simulink model "sim_main_esb_14"  (R2019b)
settings: Solver=VariableStepAuto  StartTime=0.0  StopTime=1  RelTol=1e-3
values from neighbouring files (symbols this model uses):
  C = 0.344    [KALMAN.m]    (also in main_sys.m = double( subs( C) ); main_sys_klm.m = double( subs( C) ); main_tf_0.m = [ 0 , 0  , Ks , ds , -Ks , -ds, 0 ]; main_tf_1.m = C_mes)
  Ct = double( subs( Ct) )    [main_sys.m]    (also in main_sys_klm.m; main_tf_10.m; main_tf_11.m; main_tf_12.m)
  sys_sys = ss(A,B,C,D)    [main_sys.m]    (also in main_sys_klm.m; main_tf_10.m; main_tf_11.m; main_tf_12.m = ss(A_sys,B_sys,C_sys_mod,D_sys_mod))
  Trq_mot_nom = .56    (= 0.56)    [main_cntl.m]    (also in main_sys.m; main_sys_klm.m; main_tf_10.m; main_tf_11.m)
  Tsk = .001    (= 0.001)    [main_tf_11.m]    (also in main_tf_12.m; main_tf_13.m)
  v_trq = 35e-3    (= 0.035)    [main_tf_11.m]    (also in main_tf_12.m; main_tf_13.m)
  v_vel = .1e-6    (= 1e-07)    [main_tf_11.m]    (also in main_tf_12.m; main_tf_13.m)
  w_trq = .1e-3    (= 0.0001)    [main_tf_11.m]    (also in main_tf_12.m; main_tf_13.m)
  w_vel = .15e-3    (= 0.00015)    [main_tf_11.m]    (also in main_tf_12.m; main_tf_13.m)
undefined symbols (not defined in the file or in its folder): Discrete, K_lq3, Time
libraries: ctrlSharedLib x1
settings Model: Creator=eshojaei  LastModifiedBy=eshojaei
settings DataIOCC: ReturnWorkspaceOutputs=off
settings DebuggingCC: ArithmeticOperatorsInVariantConditions=warning
settings SFSimCC: CustomCodeUndefinedFunction=UseInterfaceOnly
settings CodeAppCC: StateflowObjectComments=on

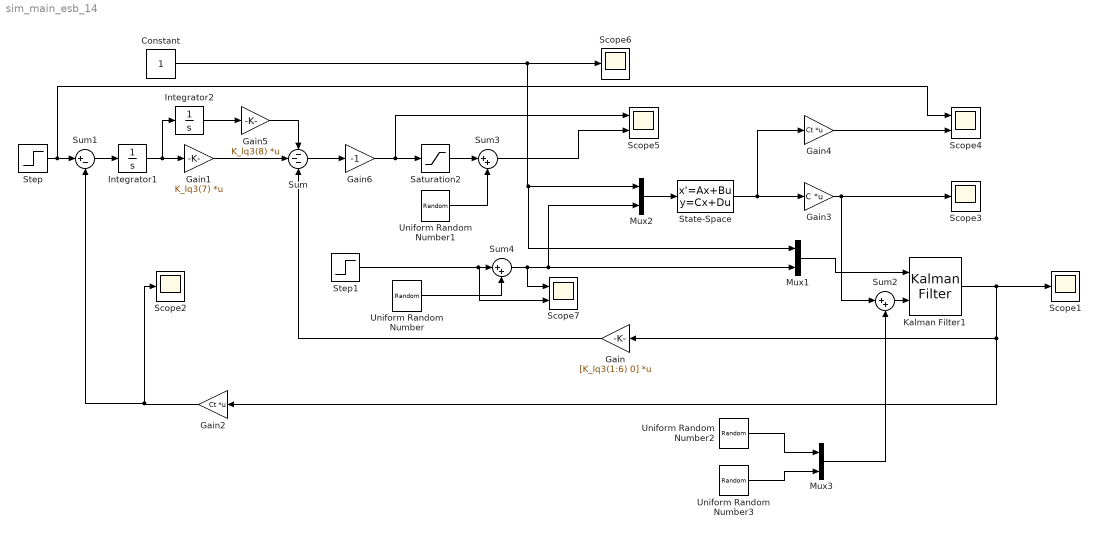
== system sim_main_esb_14 ==
  Constant : Constant
  Gain : Gain  Gain=[K_lq3(1:6) 0]  Multiplication=Matrix(K*u)
  Gain1 : Gain  Gain=K_lq3(7)  Multiplication=Matrix(K*u)
  Gain2 : Gain  Gain=Ct  Multiplication=Matrix(K*u)
  Gain3 : Gain  Gain=C  Multiplication=Matrix(K*u)
  Gain4 : Gain  Gain=Ct  Multiplication=Matrix(K*u)
  Gain5 : Gain  Gain=K_lq3(8)  Multiplication=Matrix(K*u)
  Gain6 : Gain  Gain=-1
  Integrator1 : Integrator
  Integrator2 : Integrator
  Kalman Filter1 : ctrlSharedLib/Kalman Filter  TimeDomain=Discrete-Time  UseCurrentEstimator=on  ModelSource=LTI State-Space Variable  ModelSourceVariable=ss(0.95,1,1,0,1)  A=0.95  B=1  C=1  D=0  NumberOfStates=1  NumberOfInputs=1  NumberOfOutputs=1  InitialEstimateSource=Dialog  X0=0  P0=10  UseK=off  UseGH=off  NumberOfProcessNoiseInputs=1  G=1  TimeInvariantG=on  H=0  TimeInvariantH=on  Q=0.05  TimeInvariantQ=on  R=1  TimeInvariantR=on  N=0  TimeInvariantN=on  AddInputPort=on  AddEnablePort=off  OutputEstimatedY=off  OutputP=off  Ts=-1
      settings: SourceProductBaseCode=CT
  Mux1 : Mux  Inputs=2
  Mux2 : Mux  Inputs=2
  Mux3 : Mux  Inputs=2
  Saturation2 : Saturate  UpperLimit=Trq_mot_nom * inf  LowerLimit=-Trq_mot_nom * inf
  Scope{1..3,6} (4 alike) : Scope
  Scope4 : Scope  NumInputPorts=2
  Scope5 : Scope  NumInputPorts=2
  Scope7 : Scope  NumInputPorts=2
  State-Space : StateSpace  A=sys_sys.A  B=sys_sys.B  C=sys_sys.C  D=sys_sys.D  InitialCondition=0
  Step : Step  Time=.1  After=10  SampleTime=0
  Step1 : Step  Time=.1  After=.1  SampleTime=0
  Sum : Sum  Inputs=---
  Sum1 : Sum  Inputs=|+-
  Sum2 : Sum  Inputs=|++
  Sum3 : Sum  Inputs=|++
  Sum4 : Sum  Inputs=|++
  Uniform Random Number : UniformRandomNumber  Minimum=-w_vel  Maximum=w_vel  Seed=1  SampleTime=Tsk
  Uniform Random Number1 : UniformRandomNumber  Minimum=-w_trq  Maximum=w_trq  SampleTime=Tsk
  Uniform Random Number2 : UniformRandomNumber  Minimum=-v_vel  Maximum=v_vel  SampleTime=Tsk
  Uniform Random Number3 : UniformRandomNumber  Minimum=-v_trq  Maximum=v_trq  SampleTime=Tsk
  wires:
  Step/1 -> Scope4/1, Sum1/1
  Integrator1/1 -> Integrator2/1, Gain1/1
  Gain2/1 -> Sum1/2, Scope2/1
  Sum1/1 -> Integrator1/1
  Gain3/1 -> Sum2/1, Scope3/1
  State-Space/1 -> Gain3/1, Gain4/1
  Gain4/1 -> Scope4/2
  Mux1/1 -> Kalman Filter1/1
  Mux2/1 -> State-Space/1
  Kalman Filter1/1 -> Gain2/1, Gain/1, Scope1/1
  Integrator2/1 -> Gain5/1
  Gain/1 -> Sum/3
  Gain1/1 -> Sum/2
  Gain5/1 -> Sum/1
  Sum/1 -> Gain6/1
  Gain6/1 -> Saturation2/1, Scope5/1
  Saturation2/1 -> Sum3/1
  Uniform Random Number1/1 -> Sum3/2
  Sum4/1 -> Scope7/1, Mux2/2, Mux1/2
  Uniform Random Number/1 -> Sum4/2
  Step1/1 -> Scope7/2, Sum4/1
  Uniform Random Number2/1 -> Mux3/1
  Uniform Random Number3/1 -> Mux3/2
  Sum2/1 -> Kalman Filter1/2
  Mux3/1 -> Sum2/2
  Constant/1 -> Mux1/1, Mux2/1, Scope6/1
  Sum3/1 -> Scope5/2
